simulink model "Pokus07_Display_8x8"  (Simulink 8.1)
settings: Solver=FixedStepDiscrete  StartTime=0.0  StopTime=10.0  RelTol=1e-3
libraries: simulink_extras x1, Displays_Lib x1, Computer_Library x1
settings Model: Creator=uzivatel  LastModifiedBy=uzivatel
settings DataIOCC: SignalLoggingSaveFormat=Dataset
settings OptimizationCC: ExpressionDepthLimit=128
settings DebuggingCC: FcnCallInpInsideContextMsg=EnableAllAsError
settings GRTTargetCC: CombineOutputUpdateFcns=on  GRTInterface=off

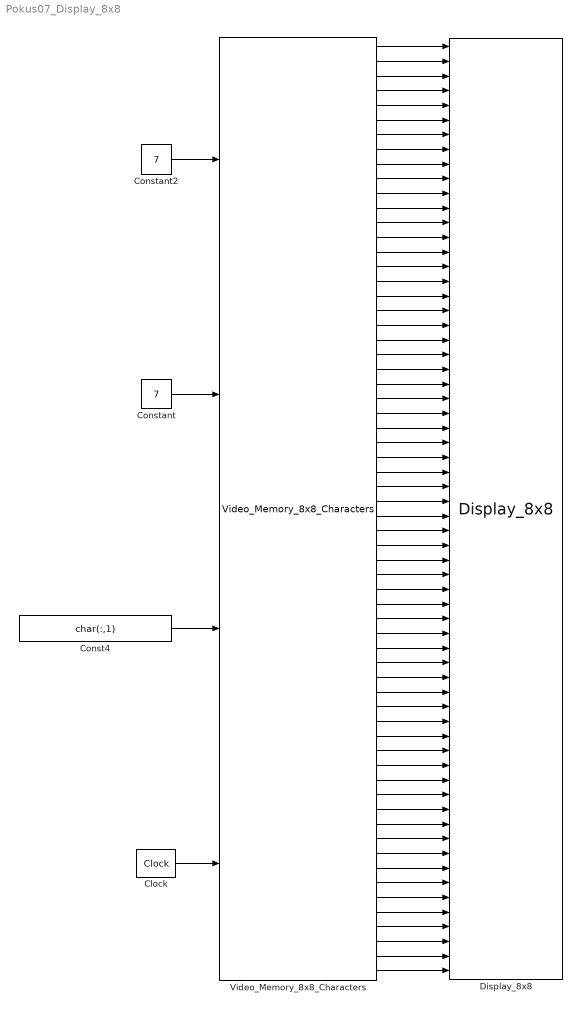
== system Pokus07_Display_8x8 ==
  Clock : simulink_extras/Flip Flops/Clock  period=1
  Const4 : Constant  Value=char(:,1)  OutDataTypeStr=uint8
  Constant : Constant  Value=7  OutDataTypeStr=uint8
  Constant2 : Constant  Value=7  OutDataTypeStr=uint8
  Display_8x8 : Displays_Lib/Displays_Lib/Display_8x8
  Video_Memory_8x8_Characters : Computer_Library/Video_Memory_8x8_Characters
  wires:
  Const4/1 -> Video_Memory_8x8_Characters/3
  Constant2/1 -> Video_Memory_8x8_Characters/1
  Constant/1 -> Video_Memory_8x8_Characters/2
  Clock/1 -> Video_Memory_8x8_Characters/4
  Video_Memory_8x8_Characters/1 -> Display_8x8/1
  Video_Memory_8x8_Characters/2 -> Display_8x8/2
  Video_Memory_8x8_Characters/3 -> Display_8x8/3
  Video_Memory_8x8_Characters/4 -> Display_8x8/4
  Video_Memory_8x8_Characters/5 -> Display_8x8/5
  Video_Memory_8x8_Characters/6 -> Display_8x8/6
  Video_Memory_8x8_Characters/7 -> Display_8x8/7
  Video_Memory_8x8_Characters/8 -> Display_8x8/8
  Video_Memory_8x8_Characters/9 -> Display_8x8/9
  Video_Memory_8x8_Characters/10 -> Display_8x8/10
  Video_Memory_8x8_Characters/11 -> Display_8x8/11
  Video_Memory_8x8_Characters/12 -> Display_8x8/12
  Video_Memory_8x8_Characters/13 -> Display_8x8/13
  Video_Memory_8x8_Characters/14 -> Display_8x8/14
  Video_Memory_8x8_Characters/15 -> Display_8x8/15
  Video_Memory_8x8_Characters/16 -> Display_8x8/16
  Video_Memory_8x8_Characters/17 -> Display_8x8/17
  Video_Memory_8x8_Characters/18 -> Display_8x8/18
  Video_Memory_8x8_Characters/19 -> Display_8x8/19
  Video_Memory_8x8_Characters/20 -> Display_8x8/20
  Video_Memory_8x8_Characters/21 -> Display_8x8/21
  Video_Memory_8x8_Characters/22 -> Display_8x8/22
  Video_Memory_8x8_Characters/23 -> Display_8x8/23
  Video_Memory_8x8_Characters/24 -> Display_8x8/24
  Video_Memory_8x8_Characters/25 -> Display_8x8/25
  Video_Memory_8x8_Characters/26 -> Display_8x8/26
  Video_Memory_8x8_Characters/27 -> Display_8x8/27
  Video_Memory_8x8_Characters/28 -> Display_8x8/28
  Video_Memory_8x8_Characters/29 -> Display_8x8/29
  Video_Memory_8x8_Characters/30 -> Display_8x8/30
  Video_Memory_8x8_Characters/31 -> Display_8x8/31
  Video_Memory_8x8_Characters/32 -> Display_8x8/32
  Video_Memory_8x8_Characters/33 -> Display_8x8/33
  Video_Memory_8x8_Characters/34 -> Display_8x8/34
  Video_Memory_8x8_Characters/35 -> Display_8x8/35
  Video_Memory_8x8_Characters/36 -> Display_8x8/36
  Video_Memory_8x8_Characters/37 -> Display_8x8/37
  Video_Memory_8x8_Characters/38 -> Display_8x8/38
  Video_Memory_8x8_Characters/39 -> Display_8x8/39
  Video_Memory_8x8_Characters/40 -> Display_8x8/40
  Video_Memory_8x8_Characters/41 -> Display_8x8/41
  Video_Memory_8x8_Characters/42 -> Display_8x8/42
  Video_Memory_8x8_Characters/43 -> Display_8x8/43
  Video_Memory_8x8_Characters/44 -> Display_8x8/44
  Video_Memory_8x8_Characters/45 -> Display_8x8/45
  Video_Memory_8x8_Characters/46 -> Display_8x8/46
  Video_Memory_8x8_Characters/47 -> Display_8x8/47
  Video_Memory_8x8_Characters/48 -> Display_8x8/48
  Video_Memory_8x8_Characters/49 -> Display_8x8/49
  Video_Memory_8x8_Characters/50 -> Display_8x8/50
  Video_Memory_8x8_Characters/51 -> Display_8x8/51
  Video_Memory_8x8_Characters/52 -> Display_8x8/52
  Video_Memory_8x8_Characters/53 -> Display_8x8/53
  Video_Memory_8x8_Characters/54 -> Display_8x8/54
  Video_Memory_8x8_Characters/55 -> Display_8x8/55
  Video_Memory_8x8_Characters/56 -> Display_8x8/56
  Video_Memory_8x8_Characters/57 -> Display_8x8/57
  Video_Memory_8x8_Characters/58 -> Display_8x8/58
  Video_Memory_8x8_Characters/59 -> Display_8x8/59
  Video_Memory_8x8_Characters/60 -> Display_8x8/60
  Video_Memory_8x8_Characters/61 -> Display_8x8/61
  Video_Memory_8x8_Characters/62 -> Display_8x8/62
  Video_Memory_8x8_Characters/63 -> Display_8x8/63
  Video_Memory_8x8_Characters/64 -> Display_8x8/64
